simulink model "ModifiedBatteryModel2"  (R2019a)
settings: Solver=VariableStepAuto  StartTime=0.0  StopTime=2500  RelTol=1e-3
libraries: nesl_utility x7, fl_lib x5
settings Model: Creator=nikos  LastModifiedBy=nikos

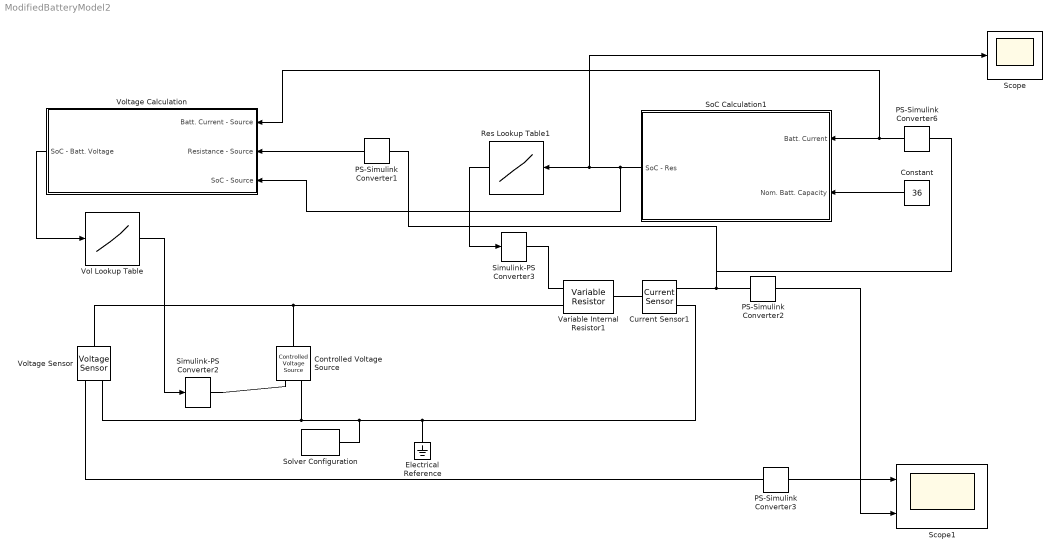
== system ModifiedBatteryModel2 ==
  Constant : Constant  Value=36
  Controlled Voltage Source : fl_lib/Electrical/Electrical Sources/Controlled Voltage Source
  Current Sensor1 : fl_lib/Electrical/Electrical Sensors/Current Sensor
  Electrical Reference : fl_lib/Electrical/Electrical Elements/Electrical Reference
  PS-Simulink Converter{1..3,6} (4 alike) : nesl_utility/PS-Simulink Converter  PhysicalDomain=network_engine_domain  SubClassName=ps_output  LeftPortType=input  RightPortType=output  PseudoPeriodic=off  Frequencies=[]  Unit=1  AffineConversion=off
  Res Lookup Table1 : Lookup_n-D  NumberOfTableDimensions=1  BreakpointsForDimension1=[0, 10, 20, 30, 40, 50, 60, 70, 80, 90, 100]  Table=[0.011448, 0.011038, 0.011281, 0.011236, 0.010959, 0.010714, 0.010698, 0.010712, 0.010917, 0.011304, 0.011603]  InternalRulePriority=Speed  RndMeth=Simplest  InputSameDT=on
  Scope : Scope
  Scope1 : Scope  NumInputPorts=2
  Simulink-PS Converter2 : nesl_utility/Simulink-PS Converter  PhysicalDomain=network_engine_domain  SubClassName=ps_input  LeftPortType=input  RightPortType=output  PseudoPeriodic=off  Frequencies=[]  NoiseDistribution=none  NoiseParameters=[]  Unit=1  AffineConversion=off  FilteringAndDerivatives=filter  SimscapeFilterOrder=1  InputFilterTimeConstant=0.001  UdotUserProvided=1
  Simulink-PS Converter3 : nesl_utility/Simulink-PS Converter  PhysicalDomain=network_engine_domain  SubClassName=ps_input  LeftPortType=input  RightPortType=output  PseudoPeriodic=off  Frequencies=[]  NoiseDistribution=none  NoiseParameters=[]  Unit=1  AffineConversion=off  FilteringAndDerivatives=zero  SimscapeFilterOrder=1  InputFilterTimeConstant=0.001  UdotUserProvided=1
  SoC Calculation1 : Subsystem
  Solver Configuration : nesl_utility/Solver Configuration  PhysicalDomain=network_engine_domain  SubClassName=solver  LeftPortType=input  RightPortType=generic  Tones=[]  Harmonics=[]  SimulateNoise=off  Profile=off  UseLocalSampling=off  EnableSwitchedLinearOptims=on  FrequencyDomain=off  UseCCode=off  RelTol=0.001  AbsTol=1e-06  MinStep=1e-09  ToWorkspace=off  RevertToSquareIcSolve=off  NumHomotopyIterations=100  PhasorMode=off  PhasorModeNumHarmonics=1  DoDC=off  ResidualTolerance=1e-09  UseLocalSolver=off  LocalSolverChoice=NE_BACKWARD_EULER_ADVANCER  LocalSolverSampleTime=0.001  DoFixedCost=off  MaxNonlinIter=3  MaxModeIter=2  LinearAlgebra=Sparse  EquationFormulation=NE_TIME_EF  DelaysMemoryBudget=1024  AutomaticFiltering=on  FilteringTimeConstant=0.001  PartitionStorageMethod=AS_NEEDED  PartitionMemoryBudget=1024  PartitionMethod=FAST
  Variable Internal Resistor1 : fl_lib/Electrical/Electrical Elements/Variable Resistor  Rmin=1 Ohm  i_specify=off  i_priority=High  i=0 A  i_nominal_specify=off  i_nominal_unit=A  i_nominal_value=1  v_specify=off  v_priority=High  v=0 V  v_nominal_specify=off  v_nominal_unit=V  v_nominal_value=1
  Vol Lookup Table : Lookup_n-D  NumberOfTableDimensions=1  BreakpointsForDimension1=[0,10,20,30,40,50,60,70,80,90,100]  Table=[35.042,35.573,36.009,36.393,36.742,37.121,37.937,38.753,39.7,40.821,41.9299999]  InternalRulePriority=Speed  RndMeth=Simplest  InputSameDT=on
  Voltage Calculation : Subsystem
  Voltage Sensor : fl_lib/Electrical/Electrical Sensors/Voltage Sensor
  wires:
  PS-Simulink Converter1/1 -> Voltage Calculation/2("Resistance - Source ")
  Res Lookup Table1/1 -> Simulink-PS Converter3/1
  SoC Calculation1/1(SoC - Res) -> Scope/1, Res Lookup Table1/1, Voltage Calculation/3(SoC - Source)
  Constant/1 -> SoC Calculation1/2("Nom. Batt. Capacity ")
  PS-Simulink Converter6/1 -> SoC Calculation1/1("Batt. Current "), Voltage Calculation/1(Batt. Current - Source)
  Vol Lookup Table/1 -> Simulink-PS Converter2/1
  Voltage Calculation/1("SoC - Batt. Voltage ") -> Vol Lookup Table/1
  PS-Simulink Converter2/1 -> Scope1/2
  PS-Simulink Converter3/1 -> Scope1/1
  connections:
  Controlled Voltage Source/LConn1 -- Voltage Sensor/LConn1 -- Variable Internal Resistor1/LConn2
  Controlled Voltage Source/RConn2 -- Voltage Sensor/RConn2 -- Solver Configuration/RConn1 -- Current Sensor1/RConn2 -- Electrical Reference/LConn1
  Current Sensor1/LConn1 -- Variable Internal Resistor1/RConn1
  Simulink-PS Converter3/RConn1 -- Variable Internal Resistor1/LConn1
  Simulink-PS Converter2/RConn1 -- Controlled Voltage Source/RConn1
  Current Sensor1/RConn1 -- PS-Simulink Converter1/LConn1 -- PS-Simulink Converter6/LConn1 -- PS-Simulink Converter2/LConn1
  Voltage Sensor/RConn1 -- PS-Simulink Converter3/LConn1

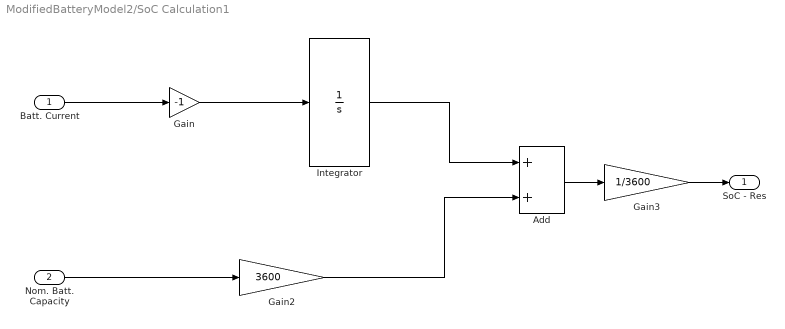
== system ModifiedBatteryModel2/SoC Calculation1 ==
  "Batt. Current " : Inport
  "Nom. Batt. Capacity " : Inport  Port=2  OutMin=0  OutMax=100
  Add : Sum
  Gain : Gain  Gain=-1
  Gain2 : Gain  Gain=3600
  Gain3 : Gain  Gain=1/3600
  Integrator : Integrator
  SoC - Res : Outport
  wires:
  "Batt. Current "/1 -> Gain/1
  Gain/1 -> Integrator/1
  "Nom. Batt. Capacity "/1 -> Gain2/1
  Gain2/1 -> Add/2
  Add/1 -> Gain3/1
  Integrator/1 -> Add/1
  Gain3/1 -> SoC - Res/1

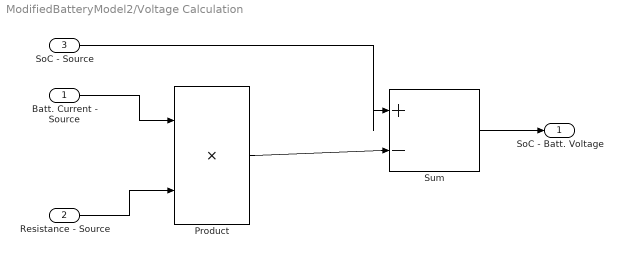
== system ModifiedBatteryModel2/Voltage Calculation ==
  Batt. Current - Source : Inport
  "Resistance - Source " : Inport  Port=2
  SoC - Source : Inport  Port=3
  Product : Product
  Sum : Sum  Inputs=|+-
  "SoC - Batt. Voltage " : Outport
  wires:
  Sum/1 -> "SoC - Batt. Voltage "/1
  SoC - Source/1 -> Sum/1
  "Resistance - Source "/1 -> Product/2
  Batt. Current - Source/1 -> Product/1
  Product/1 -> Sum/2
